simulink model "dpd_pa"  (Simulink 8.7)
settings: Solver=VariableStepDiscrete  StartTime=0.0  StopTime=hepta_dpd_pa_param.endTime  RelTol=1e-3
PreLoadFcn:
  | % Run the setup script when the model is opened
  | setup_dpd_pa;
InitFcn:
  | % Run the setup script again just before the
  | % model is run, so that any updates made
  | % after opening are applied.
  | setup_dpd_pa;
undefined symbols (not defined in the file or in its folder): AdvDSPBChannelOutDisplay, dpoly, dspba_ChannelInVis, dspba_ChannelOutVis, dspba_internal_get_channel_ports, evalAionMaskParam, hepta_dpd_pa_param, latency, value
libraries: DSPBAPrim x159, DSPBABase x6, DSPBAAvalonST x2, DSPBAUtilities x1
(part 1 of 2)
Description:
  | DSP Builder Advanced Template for Template Design implementing Primitive Subsystems
settings Model: Creator=mjervis  LastModifiedBy=5g
settings DataIOCC: SignalLoggingSaveFormat=ModelDataLogs
settings OptimizationCC: ExpressionDepthLimit=2147483647
settings DebuggingCC: SolverPrmCheckMsg=warning  InheritedTsInSrcMsg=none  IntegerOverflowMsg=none  FcnCallInpInsideContextMsg=UseLocalSettings  StateNameClashWarn=warning  IntegerSaturationMsg=none
settings GRTTargetCC: CombineOutputUpdateFcns=off  GRTInterface=on
settings ConfigComp: CovSFcnEnable=off

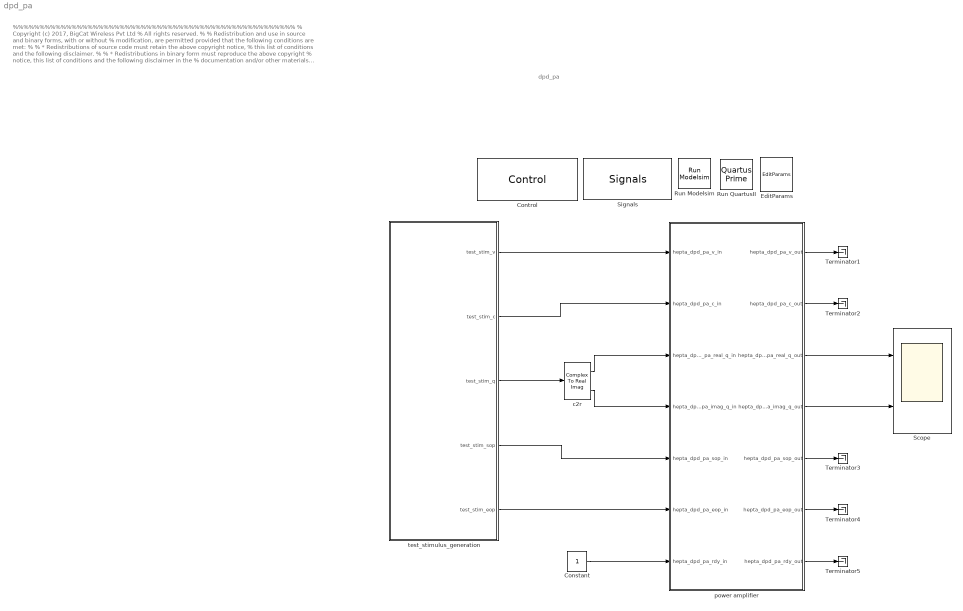
== system dpd_pa ==
  note: %%%%%%%%%%%%%%%%%%%%%%%%%%%%%%%%%%%%%%%%%%%%%%%%%%%%%
      |  % Copyright (c) 2017, BigCat Wireless Pvt Ltd
      |  % All rights reserved.
      |  %
      |  % Redistribution and use in source and binary forms, with or without
      |  % modification, are permitted provided that the following conditions are met:
      |  %
      |  %     * Redistributions of source code must retain the above copyright notice,
      |  %       this list of conditions and the following disclaimer.
      |  %
      |  %     * Redistributions in binary form must reproduce the above copyright
      |  %       notice, this list of conditions and the following disclaimer in the
      |  %       documentation and/or other materials provided with the distribution.
      |  %
      |  %     * Neither the name of the copyright holder nor the names of its contributors
      |  %       may be used to endorse or promote products derived from this software
      |  %       without specific prior written permission.
      |  %
      |  %
      |  %
      |  % THIS SOFTWARE IS PROVIDED BY THE COPYRIGHT HOLDERS AND CONTRIBUTORS "AS IS"
      |  % AND ANY EXPRESS OR IMPLIED WARRANTIES, INCLUDING, BUT NOT LIMITED TO, THE
      |  % IMPLIED WARRANTIES OF MERCHANTABILITY AND FITNESS FOR A PARTICULAR PURPOSE ARE
      |  % DISCLAIMED. IN NO EVENT SHALL THE COPYRIGHT HOLDER OR CONTRIBUTORS BE LIABLE
      |  % FOR ANY DIRECT, INDIRECT, INCIDENTAL, SPECIAL, EXEMPLARY, OR CONSEQUENTIAL
      |  % DAMAGES (INCLUDING, BUT NOT LIMITED TO, PROCUREMENT OF SUBSTITUTE GOODS OR
      |  % SERVICES; LOSS OF USE, DATA, OR PROFITS; OR BUSINESS INTERRUPTION) HOWEVER
      |  % CAUSED AND ON ANY THEORY OF LIABILITY, WHETHER IN CONTRACT, STRICT LIABILITY,
      |  % OR TORT (INCLUDING NEGLIGENCE OR OTHERWISE) ARISING IN ANY WAY OUT OF THE USE
      |  % OF THIS SOFTWARE, EVEN IF ADVISED OF THE POSSIBILITY OF SUCH DAMAGE.
      |  %
      |   %%%%%%%%%%%%%%%%%%%%%%%%%%%%%%%%%%%%%%%%%%%%%%%%%%%%%
  note: dpd_pa
  Constant : Constant  OutDataTypeStr=boolean
  Control : DSPBABase/Control  generate=on  language=VHDL  destination=./rtl  make_full_path=off  path_is_relative=on  autotestbench=on  signaldepth=2  coveragetestbench=on  logs=off  spacewidth=2  spacenum=1  addrwidth=13  datawidth=32  dataendian=Big Endian  hierarchicalnames=off  ramThresholdBits=-1  distRamThresholdBits=-1  mlabThresholdBits=-1  hardMultiplierThresholdLuts=-1  version=20090407  errorOnChanMismatch=1  errorOnGPIOMismatch=0  importModelsimResults=0  cycleAccurate=off  reinterpretCastMult=off  paramFile=dpd_pa_params.xml
  EditParams : DSPBABase/EditParams  version=20090407
  Run Modelsim : DSPBABase/Run Modelsim  version=20090407
  "Run QuartusII " : DSPBABase/Quartus Prime  version=20090407
  Scope : Scope  NumInputPorts=2
  Signals : DSPBABase/Signals  clk=clk  freq=hepta_dpd_pa_param.ClockRate  margin=hepta_dpd_pa_param.ClockMargin  rst=areset  rstactive=High  bus=bus  enbusclock=on  busfreq=61.44  bussync=on  version=20090407
  Terminator{1..5} (5 alike) : Terminator
  c2r : ComplexToRealImag
  power amplifier : Subsystem
  test_stimulus_generation : Subsystem
  wires:
  test_stimulus_generation/1(test_stim_v) -> power amplifier/1(hepta_dpd_pa_v_in)
  test_stimulus_generation/2(test_stim_c) -> power amplifier/2(hepta_dpd_pa_c_in)
  test_stimulus_generation/3(test_stim_q) -> c2r/1
  c2r/1 -> power amplifier/3(hepta_dpd_pa_real_q_in)
  c2r/2 -> power amplifier/4(hepta_dpd_pa_imag_q_in)
  Constant/1 -> power amplifier/7(hepta_dpd_pa_rdy_in)
  power amplifier/1(hepta_dpd_pa_v_out) -> Terminator1/1
  power amplifier/2(hepta_dpd_pa_c_out) -> Terminator2/1
  power amplifier/5(hepta_dpd_pa_sop_out) -> Terminator3/1
  power amplifier/6(hepta_dpd_pa_eop_out) -> Terminator4/1
  power amplifier/7(hepta_dpd_pa_rdy_out) -> Terminator5/1
  power amplifier/3(hepta_dpd_pa_real_q_out) -> Scope/1
  power amplifier/4(hepta_dpd_pa_imag_q_out) -> Scope/2
  test_stimulus_generation/5(test_stim_eop) -> power amplifier/6(hepta_dpd_pa_eop_in)
  test_stimulus_generation/4(test_stim_sop) -> power amplifier/5(hepta_dpd_pa_sop_in)

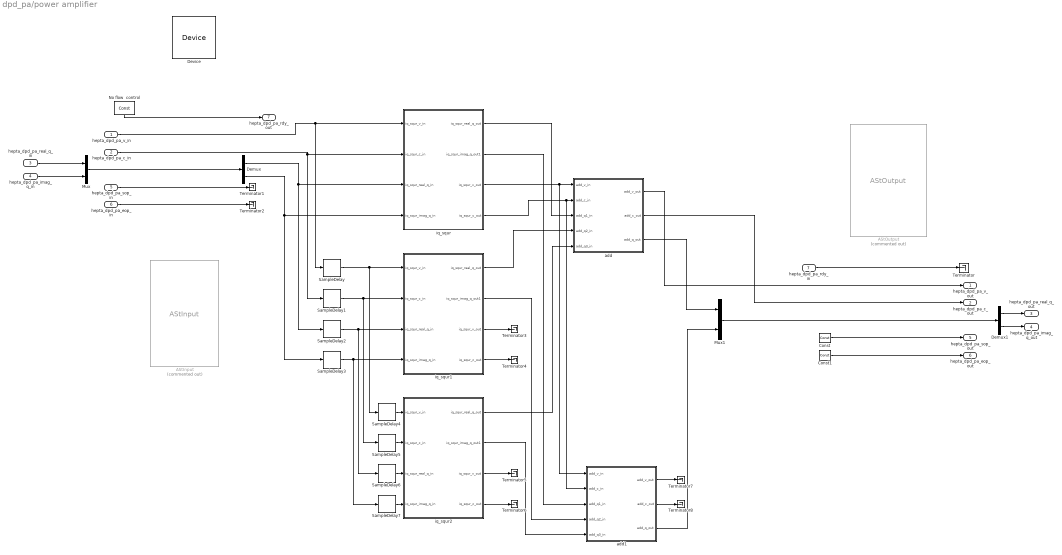
== system dpd_pa/power amplifier ==
  hepta_dpd_pa_v_in : Inport
  hepta_dpd_pa_c_in : Inport  Port=2
  hepta_dpd_pa_real_q_in : Inport  Port=3
  hepta_dpd_pa_imag_q_in : Inport  Port=4
  hepta_dpd_pa_sop_in : Inport  Port=5
  hepta_dpd_pa_eop_in : Inport  Port=6
  hepta_dpd_pa_rdy_in : Inport  Port=7
  AStInput : DSPBAAvalonST/AStInput  Commented=on
      link override BasicAvInput/sopOvrflw/setOrRst1: omode=Inherit via internal rule  otype=ufix(1)  scale=2^0
      link override ChannelOut: value=3  latency=1
  AStOutput : DSPBAAvalonST/AStOutput  Commented=on  fifo_setup=[12 4 8]
      link override ChannelOut: value=4  latency=0
  Const : DSPBAPrim/Const  primtype=const  nInputs=0  nOutputs=1  omode=boolean  otype=sfix(16)  scale=2^-15  rndmethod=Unbiased  factor=1  satmethod=Symmetric  shift_vec=[0 1 2 -1]  value=0  inPortNames=['+'; '+';]  outPortNames=[' ']  dspbaimage=dspba_prim.jpg  text=fprintf('%s', num2str(value));  style=Optimised  visibilities=8 + 1024  floatPrecision=float32_m23  version=20120820
  Const1 : DSPBAPrim/Const  primtype=const  nInputs=0  nOutputs=1  omode=boolean  otype=sfix(16)  scale=2^-15  rndmethod=Unbiased  factor=1  satmethod=Symmetric  shift_vec=[0 1 2 -1]  value=0  inPortNames=['+'; '+';]  outPortNames=[' ']  dspbaimage=dspba_prim.jpg  text=fprintf('%s', num2str(value));  style=Optimised  visibilities=8 + 1024  floatPrecision=float32_m23  version=20120820
  Demux : Demux  Outputs=2
  Demux1 : Demux  Outputs=2
  Device : DSPBABase/Device  family=Arria 10  deviceMember=Arria 10  stratix4device=Stratix IV GX  hardcopy4device=HardCopy IV E  stratix5device=Stratix V GX  device=10AS066N2F40I1SGES  speed=1  stratixSpeed=-5  stratix2Speed=-3  stratix3Speed=-3  stratix4gxSpeed=-2  stratix4gtSpeed=-1  cyclone2Speed=-6  cyclone3Speed=-7  arria2Speed=-4  cyclone4eSpeed=-8  stratix5Speed=-3  arria5Speed=-4  arriaSpeed=-6  cyclone3lsSpeed=-7  cyclone5Speed=-6  arria2gzSpeed=-3  nightFurySpeed=-2  ecp2Speed=-7  hardcopycompat=off  version=20140217  max10flashmode=off  max10nomeminit=off
  Mux : Mux  Inputs=2
  Mux1 : Mux  Inputs=2
  No flow  control : DSPBAPrim/Const  primtype=const  nInputs=0  nOutputs=1  omode=Inherit via internal rule  otype=sfix(16)  scale=2^-15  rndmethod=Unbiased  factor=1  satmethod=Symmetric  shift_vec=[0 1 2 -1]  value=1  inPortNames=['+'; '+';]  outPortNames=[' ']  dspbaimage=dspba_prim.jpg  text=fprintf('%s', num2str(value));  style=Optimised  visibilities=8 + 1024  floatPrecision=float32_m23  version=20120820
  SampleDelay{,1..7} (8 alike) : DSPBAPrim/SampleDelay  primtype=sampdelay  nInputs=1  nOutputs=1  omode=Inherit via internal rule  otype=sfix(16)  scale=2^-15  rndmethod=Unbiased  factor=1  satmethod=Symmetric  shift_vec=[0 1 2 -1]  value=1  inPortNames=[' '; ' ';]  outPortNames=[' ']  dspbaimage=dspba_prim.jpg  text=dpoly(1, eye(1,value+1), 'z')  style=Optimised  visibilities=8 + 1024 + 2^17 + 2^18  flexible=off  slackgroup=0  augmented=0  version=20090407  advOptions=[]
  Terminator{,1..8} (9 alike) : Terminator
  add : Subsystem
  add1 : Subsystem
  iq_squr : Subsystem
  iq_squr1 : Subsystem
  iq_squr2 : Subsystem
  hepta_dpd_pa_v_out : Outport
  hepta_dpd_pa_c_out : Outport  Port=2
  hepta_dpd_pa_real_q_out : Outport  Port=3
  hepta_dpd_pa_imag_q_out : Outport  Port=4
  hepta_dpd_pa_sop_out : Outport  Port=5
  hepta_dpd_pa_eop_out : Outport  Port=6
  hepta_dpd_pa_rdy_out : Outport  Port=7
  wires:
  No flow  control/1 -> hepta_dpd_pa_rdy_out/1
  hepta_dpd_pa_real_q_in/1 -> Mux/1
  hepta_dpd_pa_imag_q_in/1 -> Mux/2
  Mux/1 -> Demux/1
  Demux/2 -> SampleDelay3/1, iq_squr/4(iq_squr_imag_q_in)
  add/1(add_v_out) -> hepta_dpd_pa_v_out/1
  add/2(add_c_out) -> hepta_dpd_pa_c_out/1
  Const/1 -> hepta_dpd_pa_sop_out/1
  Const1/1 -> hepta_dpd_pa_eop_out/1
  hepta_dpd_pa_rdy_in/1 -> Terminator/1
  Mux1/1 -> Demux1/1
  Demux1/2 -> hepta_dpd_pa_imag_q_out/1
  Demux1/1 -> hepta_dpd_pa_real_q_out/1
  hepta_dpd_pa_sop_in/1 -> Terminator1/1
  hepta_dpd_pa_eop_in/1 -> Terminator2/1
  hepta_dpd_pa_v_in/1 -> SampleDelay/1, iq_squr/1(iq_squr_v_in)
  Demux/1 -> SampleDelay2/1, iq_squr/3(iq_squr_real_q_in)
  hepta_dpd_pa_c_in/1 -> SampleDelay1/1, iq_squr/2(iq_squr_c_in)
  SampleDelay/1 -> iq_squr1/1(iq_squr_v_in), SampleDelay4/1
  SampleDelay1/1 -> iq_squr1/2(iq_squr_c_in), SampleDelay5/1
  SampleDelay2/1 -> iq_squr1/3(iq_squr_real_q_in), SampleDelay6/1
  SampleDelay3/1 -> iq_squr1/4(iq_squr_imag_q_in), SampleDelay7/1
  SampleDelay4/1 -> iq_squr2/1(iq_squr_v_in)
  SampleDelay5/1 -> iq_squr2/2(iq_squr_c_in)
  SampleDelay6/1 -> iq_squr2/3(iq_squr_real_q_in)
  SampleDelay7/1 -> iq_squr2/4(iq_squr_imag_q_in)
  iq_squr/3(iq_squr_v_out) -> add1/1(add_v_in), add/1(add_v_in)
  iq_squr/4(iq_squr_c_out) -> add1/2(add_c_in), add/2(add_c_in)
  iq_squr/1(iq_squr_real_q_out) -> add/3(add_q1_in)
  iq_squr1/1(iq_squr_real_q_out) -> add/4(add_q2_in)
  iq_squr2/1(iq_squr_real_q_out) -> add/5(add_q3_in)
  iq_squr2/2(iq_squr_imag_q_out1) -> add1/5(add_q3_in)
  iq_squr1/2(iq_squr_imag_q_out1) -> add1/4(add_q2_in)
  iq_squr/2(iq_squr_imag_q_out1) -> add1/3(add_q1_in)
  add/3(add_q_out) -> Mux1/1
  add1/3(add_q_out) -> Mux1/2
  iq_squr1/3(iq_squr_v_out) -> Terminator3/1
  iq_squr1/4(iq_squr_c_out) -> Terminator4/1
  iq_squr2/3(iq_squr_v_out) -> Terminator5/1
  iq_squr2/4(iq_squr_c_out) -> Terminator6/1
  add1/1(add_v_out) -> Terminator7/1
  add1/2(add_c_out) -> Terminator8/1

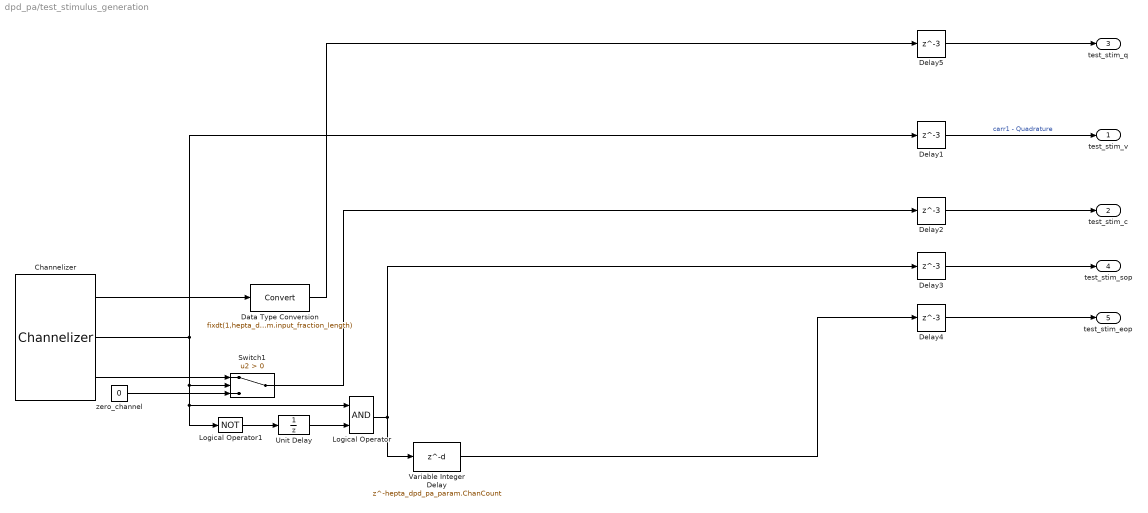
== system dpd_pa/test_stimulus_generation ==
  Channelizer : DSPBAUtilities/Channelizer  data_input=hepta_dpd_pa_param.inputdata1  folding=hepta_dpd_pa_param.Period  samples_valid=1  samples_idle=0  sample_time=hepta_dpd_pa_param.SampleTime
  Data Type Conversion : DataTypeConversion  OutDataTypeStr=fixdt(1,hepta_dpd_pa_param.input_word_length,hepta_dpd_pa_param.input_fraction_length)  SaturateOnIntegerOverflow=on
  Delay{1..4} (4 alike) : Delay  DelayLength=3  InitialCondition=0
  Delay5 : Delay  DelayLength=3  InitialCondition=0  InputProcessing=Inherited
  Logical Operator : Logic  AllPortsSameDT=off  OutDataTypeStr=boolean
  Logical Operator1 : Logic  Operator=NOT  AllPortsSameDT=off  OutDataTypeStr=boolean
  Switch1 : Switch  Criteria=u2 > Threshold
  Unit Delay : UnitDelay  SampleTime=-1
  Variable Integer Delay : Delay  DelayLength=hepta_dpd_pa_param.ChanCount  InputProcessing=Inherited
  zero_channel : Constant  Value=0  OutDataTypeStr=uint8
  test_stim_v : Outport
  test_stim_c : Outport  Port=2
  test_stim_q : Outport  Port=3
  test_stim_sop : Outport  Port=4
  test_stim_eop : Outport  Port=5
  wires:
  Channelizer/3 -> Switch1/1
  Logical Operator1/1 -> Unit Delay/1
  Channelizer/1 -> Data Type Conversion/1
  Logical Operator/1 -> Variable Integer Delay/1, Delay3/1
  zero_channel/1 -> Switch1/3
  Unit Delay/1 -> Logical Operator/2
  Channelizer/2 -> Logical Operator/1, Logical Operator1/1, Switch1/2, Delay1/1
  Switch1/1 -> Delay2/1
  Variable Integer Delay/1 -> Delay4/1
  Delay2/1 -> test_stim_c/1
  Delay3/1 -> test_stim_sop/1
  Delay4/1 -> test_stim_eop/1
  Delay1/1 -> test_stim_v/1  "carr1 - Quadrature"
  Data Type Conversion/1 -> Delay5/1
  Delay5/1 -> test_stim_q/1

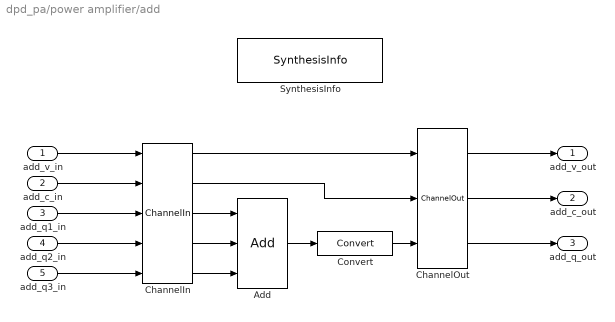
== system dpd_pa/power amplifier/add ==
  add_v_in : Inport
  add_c_in : Inport  Port=2
  add_q1_in : Inport  Port=3
  add_q2_in : Inport  Port=4
  add_q3_in : Inport  Port=5
  Add : DSPBAPrim/Add  primtype=add  nInputs=evalAionMaskParam(gcb,'value',1)  nOutputs=1  omode=Inherit via internal rule with word growth  otype=sfix(16)  scale=2^-15  rndmethod=Unbiased  factor=1  satmethod=Symmetric  shift_vec=[0 1 2 -1]  value=3  inPortNames=[' '; ' ';]  outPortNames=[' ']  dspbaimage=dspba_prim.jpg  text=fprintf('+');  style=Optimised  visibilities=1032+2^17+2^18+2^19  genFPC=off  floatRounding=correct  advOptions=[]  version=20130821
  ChannelIn : DSPBAPrim/ChannelIn  primtype=channelin  nInputs=dspba_internal_get_channel_ports(gcb)  nOutputs=dspba_internal_get_channel_ports(gcb)  omode=Inherit via internal rule  otype=sfix(16)  scale=2^-15  rndmethod=Unbiased  factor=1  satmethod=Symmetric  shift_vec=[0 1 2 -1]  value=3  inPortNames=['v'; 'c'; '0'; '1'; '2'; '3'; '4'; '5'; '6'; '7'; '8'; '9'; 'A'; 'B'; 'D'; 'E'; 'F'; 'G'; 'H'; 'I'; 'J'; 'K'; 'L'; 'M'; 'N'; 'O'; 'P'; 'Q'; 'R'; 'S'; 'T'; 'U'; 'W'; 'X'; 'Y'; 'Z']  outPortNames=['v'; 'c'; '0'; '1'; '2'; '3'; '4'; '5'; '6'; '7'; '8'; '9'; 'A'; 'B'; 'D'; 'E'; 'F'; 'G'; 'H'; 'I'; 'J'; 'K'; 'L'; 'M'; 'N'; 'O'; 'P'; 'Q'; 'R'; 'S'; 'T'; 'U'; 'W'; 'X'; 'Y'; 'Z']  dspbaimage=dspba_prim.jpg  text=fprintf('In');  style=Optimised  dataSignals=3  foldingEnabled=off  channels=1  sampleRate=200  packetBeginPresent=off  packetBeginEnabled=off  visibilities=dspba_ChannelInVis(gcb)  latencyCorrection=0  version=20141013
  ChannelOut : DSPBAPrim/ChannelOut  primtype=channelout  nInputs=dspba_internal_get_channel_ports(gcb)  nOutputs=dspba_internal_get_channel_ports(gcb)  omode=Inherit via internal rule  otype=sfix(16)  scale=2^-15  rndmethod=Unbiased  factor=1  satmethod=Symmetric  shift_vec=[0 1 2 -1]  value=1  inPortNames=['v'; 'c'; '0'; '1'; '2'; '3'; '4'; '5'; '6'; '7'; '8'; '9'; 'A'; 'B'; 'D'; 'E'; 'F'; 'G'; 'H'; 'I'; 'J'; 'K'; 'L'; 'M'; 'N'; 'O'; 'P'; 'Q'; 'R'; 'S'; 'T'; 'U'; 'W'; 'X'; 'Y'; 'Z']  outPortNames=['v'; 'c'; '0'; '1'; '2'; '3'; '4'; '5'; '6'; '7'; '8'; '9'; 'A'; 'B'; 'D'; 'E'; 'F'; 'G'; 'H'; 'I'; 'J'; 'K'; 'L'; 'M'; 'N'; 'O'; 'P'; 'Q'; 'R'; 'S'; 'T'; 'U'; 'W'; 'X'; 'Y'; 'Z']  dspbaimage=dspba_prim.jpg  text=fprintf('Out%s', AdvDSPBChannelOutDisplay(latency));  style=Optimised  dataSignals=1  foldingEnabled=off  channels=1  sampleRate=200  packetBeginPresent=off  packetBeginEnabled=off  visibilities=dspba_ChannelOutVis(gcb)  latency=0  latencyCorrection=0  version=20141013
  Convert : DSPBAPrim/Convert  primtype=convert  nInputs=1  nOutputs=1  omode=Specify via dialog  otype=sfix(16)  scale=2^-15  rndmethod=Unbiased  factor=1  satmethod=None  shift_vec=[0 1 2 -1]  value=round([0:255]/17)  inPortNames=[' '; ' ';]  outPortNames=[' '; 'c']  dspbaimage=dspba_prim.jpg  text=fprintf('convert');  style=Optimised  visibilities=8+64+256+2^17  clipdetect=off  floatPrecision=float32_m23  advOptions=[]  version=20130211
  SynthesisInfo : DSPBAPrim/SynthesisInfo  primtype=synthinfo  nInputs=0  nOutputs=0  omode=Inherit via internal rule  otype=sfix(16)  scale=2^-15  rndmethod=Truncate  factor=1  satmethod=Symmetric  shift_vec=[0 1 2 -1]  value=99  inPortNames=[' '; ' ';]  outPortNames=[' ']  dspbaimage=dspba_prim_ctrl.jpg  text=fprintf('Style=%s', style);  style=Scheduled  visibilities=2^15+2^17+2^18+2^19  constraintInUse=off  constraintRelation=>  constraintLimit=2  bitAccurate=off  version=20150220
  add_v_out : Outport
  add_c_out : Outport  Port=2
  add_q_out : Outport  Port=3
  wires:
  ChannelIn/1 -> ChannelOut/1
  add_c_in/1 -> ChannelIn/2
  add_q1_in/1 -> ChannelIn/3
  add_v_in/1 -> ChannelIn/1
  add_q2_in/1 -> ChannelIn/4
  add_q3_in/1 -> ChannelIn/5
  ChannelIn/2 -> ChannelOut/2
  ChannelOut/2 -> add_c_out/1
  Add/1 -> Convert/1
  ChannelOut/1 -> add_v_out/1
  ChannelOut/3 -> add_q_out/1
  ChannelIn/3 -> Add/1
  ChannelIn/4 -> Add/2
  ChannelIn/5 -> Add/3
  Convert/1 -> ChannelOut/3

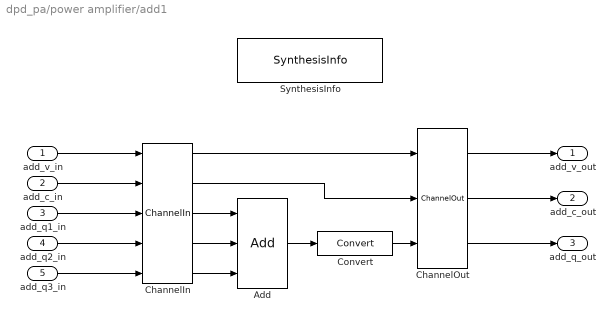
== system dpd_pa/power amplifier/add1 ==
  add_v_in : Inport
  add_c_in : Inport  Port=2
  add_q1_in : Inport  Port=3
  add_q2_in : Inport  Port=4
  add_q3_in : Inport  Port=5
  Add : DSPBAPrim/Add  primtype=add  nInputs=evalAionMaskParam(gcb,'value',1)  nOutputs=1  omode=Inherit via internal rule with word growth  otype=sfix(16)  scale=2^-15  rndmethod=Unbiased  factor=1  satmethod=Symmetric  shift_vec=[0 1 2 -1]  value=3  inPortNames=[' '; ' ';]  outPortNames=[' ']  dspbaimage=dspba_prim.jpg  text=fprintf('+');  style=Optimised  visibilities=1032+2^17+2^18+2^19  genFPC=off  floatRounding=correct  advOptions=[]  version=20130821
  ChannelIn : DSPBAPrim/ChannelIn  primtype=channelin  nInputs=dspba_internal_get_channel_ports(gcb)  nOutputs=dspba_internal_get_channel_ports(gcb)  omode=Inherit via internal rule  otype=sfix(16)  scale=2^-15  rndmethod=Unbiased  factor=1  satmethod=Symmetric  shift_vec=[0 1 2 -1]  value=3  inPortNames=['v'; 'c'; '0'; '1'; '2'; '3'; '4'; '5'; '6'; '7'; '8'; '9'; 'A'; 'B'; 'D'; 'E'; 'F'; 'G'; 'H'; 'I'; 'J'; 'K'; 'L'; 'M'; 'N'; 'O'; 'P'; 'Q'; 'R'; 'S'; 'T'; 'U'; 'W'; 'X'; 'Y'; 'Z']  outPortNames=['v'; 'c'; '0'; '1'; '2'; '3'; '4'; '5'; '6'; '7'; '8'; '9'; 'A'; 'B'; 'D'; 'E'; 'F'; 'G'; 'H'; 'I'; 'J'; 'K'; 'L'; 'M'; 'N'; 'O'; 'P'; 'Q'; 'R'; 'S'; 'T'; 'U'; 'W'; 'X'; 'Y'; 'Z']  dspbaimage=dspba_prim.jpg  text=fprintf('In');  style=Optimised  dataSignals=3  foldingEnabled=off  channels=1  sampleRate=200  packetBeginPresent=off  packetBeginEnabled=off  visibilities=dspba_ChannelInVis(gcb)  latencyCorrection=0  version=20141013
  ChannelOut : DSPBAPrim/ChannelOut  primtype=channelout  nInputs=dspba_internal_get_channel_ports(gcb)  nOutputs=dspba_internal_get_channel_ports(gcb)  omode=Inherit via internal rule  otype=sfix(16)  scale=2^-15  rndmethod=Unbiased  factor=1  satmethod=Symmetric  shift_vec=[0 1 2 -1]  value=1  inPortNames=['v'; 'c'; '0'; '1'; '2'; '3'; '4'; '5'; '6'; '7'; '8'; '9'; 'A'; 'B'; 'D'; 'E'; 'F'; 'G'; 'H'; 'I'; 'J'; 'K'; 'L'; 'M'; 'N'; 'O'; 'P'; 'Q'; 'R'; 'S'; 'T'; 'U'; 'W'; 'X'; 'Y'; 'Z']  outPortNames=['v'; 'c'; '0'; '1'; '2'; '3'; '4'; '5'; '6'; '7'; '8'; '9'; 'A'; 'B'; 'D'; 'E'; 'F'; 'G'; 'H'; 'I'; 'J'; 'K'; 'L'; 'M'; 'N'; 'O'; 'P'; 'Q'; 'R'; 'S'; 'T'; 'U'; 'W'; 'X'; 'Y'; 'Z']  dspbaimage=dspba_prim.jpg  text=fprintf('Out%s', AdvDSPBChannelOutDisplay(latency));  style=Optimised  dataSignals=1  foldingEnabled=off  channels=1  sampleRate=200  packetBeginPresent=off  packetBeginEnabled=off  visibilities=dspba_ChannelOutVis(gcb)  latency=0  latencyCorrection=0  version=20141013
  Convert : DSPBAPrim/Convert  primtype=convert  nInputs=1  nOutputs=1  omode=Specify via dialog  otype=sfix(16)  scale=2^-15  rndmethod=Unbiased  factor=1  satmethod=None  shift_vec=[0 1 2 -1]  value=round([0:255]/17)  inPortNames=[' '; ' ';]  outPortNames=[' '; 'c']  dspbaimage=dspba_prim.jpg  text=fprintf('convert');  style=Optimised  visibilities=8+64+256+2^17  clipdetect=off  floatPrecision=float32_m23  advOptions=[]  version=20130211
  SynthesisInfo : DSPBAPrim/SynthesisInfo  primtype=synthinfo  nInputs=0  nOutputs=0  omode=Inherit via internal rule  otype=sfix(16)  scale=2^-15  rndmethod=Truncate  factor=1  satmethod=Symmetric  shift_vec=[0 1 2 -1]  value=99  inPortNames=[' '; ' ';]  outPortNames=[' ']  dspbaimage=dspba_prim_ctrl.jpg  text=fprintf('Style=%s', style);  style=Scheduled  visibilities=2^15+2^17+2^18+2^19  constraintInUse=off  constraintRelation=>  constraintLimit=2  bitAccurate=off  version=20150220
  add_v_out : Outport
  add_c_out : Outport  Port=2
  add_q_out : Outport  Port=3
  wires:
  ChannelIn/1 -> ChannelOut/1
  add_c_in/1 -> ChannelIn/2
  add_q1_in/1 -> ChannelIn/3
  add_v_in/1 -> ChannelIn/1
  add_q2_in/1 -> ChannelIn/4
  add_q3_in/1 -> ChannelIn/5
  ChannelIn/2 -> ChannelOut/2
  ChannelOut/2 -> add_c_out/1
  Add/1 -> Convert/1
  ChannelOut/1 -> add_v_out/1
  ChannelOut/3 -> add_q_out/1
  ChannelIn/3 -> Add/1
  ChannelIn/4 -> Add/2
  ChannelIn/5 -> Add/3
  Convert/1 -> ChannelOut/3

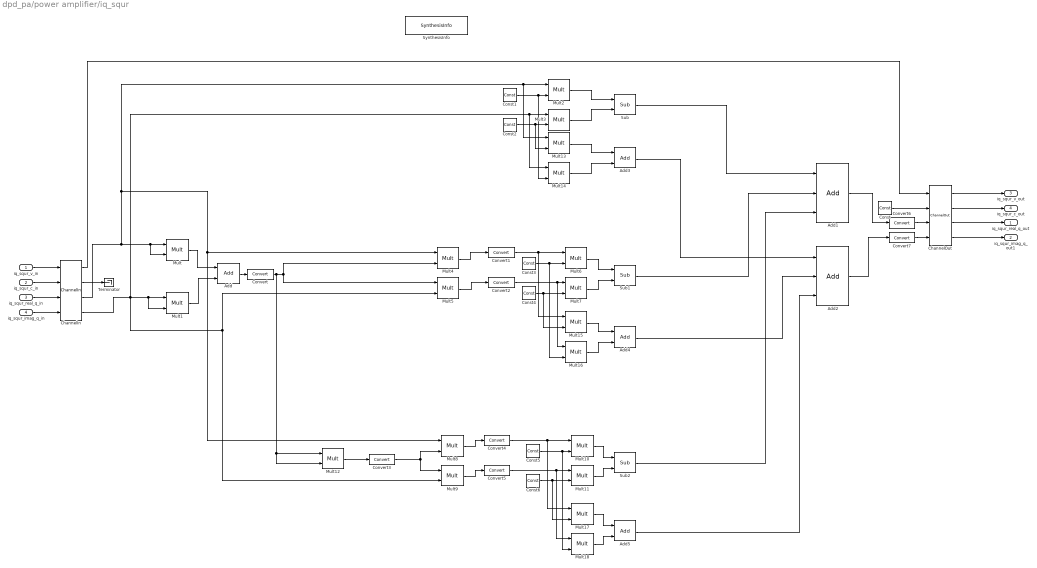
== system dpd_pa/power amplifier/iq_squr ==
  iq_squr_v_in : Inport
  iq_squr_c_in : Inport  Port=2
  iq_squr_real_q_in : Inport  Port=3
  iq_squr_imag_q_in : Inport  Port=4
  Add{,3..5} (4 alike) : DSPBAPrim/Add  primtype=add  nInputs=evalAionMaskParam(gcb,'value',1)  nOutputs=1  omode=Inherit via internal rule with word growth  otype=sfix(16)  scale=2^-15  rndmethod=Unbiased  factor=1  satmethod=Symmetric  shift_vec=[0 1 2 -1]  value=2  inPortNames=[' '; ' ';]  outPortNames=[' ']  dspbaimage=dspba_prim.jpg  text=fprintf('+');  style=Optimised  visibilities=1032+2^17+2^18+2^19  genFPC=off  floatRounding=correct  advOptions=[]  version=20130821
  Add1 : DSPBAPrim/Add  primtype=add  nInputs=evalAionMaskParam(gcb,'value',1)  nOutputs=1  omode=Inherit via internal rule with word growth  otype=sfix(16)  scale=2^-15  rndmethod=Unbiased  factor=1  satmethod=Symmetric  shift_vec=[0 1 2 -1]  value=3  inPortNames=[' '; ' ';]  outPortNames=[' ']  dspbaimage=dspba_prim.jpg  text=fprintf('+');  style=Optimised  visibilities=1032+2^17+2^18+2^19  genFPC=off  floatRounding=correct  advOptions=[]  version=20130821
  Add2 : DSPBAPrim/Add  primtype=add  nInputs=evalAionMaskParam(gcb,'value',1)  nOutputs=1  omode=Inherit via internal rule with word growth  otype=sfix(16)  scale=2^-15  rndmethod=Unbiased  factor=1  satmethod=Symmetric  shift_vec=[0 1 2 -1]  value=3  inPortNames=[' '; ' ';]  outPortNames=[' ']  dspbaimage=dspba_prim.jpg  text=fprintf('+');  style=Optimised  visibilities=1032+2^17+2^18+2^19  genFPC=off  floatRounding=correct  advOptions=[]  version=20130821
  ChannelIn : DSPBAPrim/ChannelIn  primtype=channelin  nInputs=dspba_internal_get_channel_ports(gcb)  nOutputs=dspba_internal_get_channel_ports(gcb)  omode=Inherit via internal rule  otype=sfix(16)  scale=2^-15  rndmethod=Unbiased  factor=1  satmethod=Symmetric  shift_vec=[0 1 2 -1]  value=2  inPortNames=['v'; 'c'; '0'; '1'; '2'; '3'; '4'; '5'; '6'; '7'; '8'; '9'; 'A'; 'B'; 'D'; 'E'; 'F'; 'G'; 'H'; 'I'; 'J'; 'K'; 'L'; 'M'; 'N'; 'O'; 'P'; 'Q'; 'R'; 'S'; 'T'; 'U'; 'W'; 'X'; 'Y'; 'Z']  outPortNames=['v'; 'c'; '0'; '1'; '2'; '3'; '4'; '5'; '6'; '7'; '8'; '9'; 'A'; 'B'; 'D'; 'E'; 'F'; 'G'; 'H'; 'I'; 'J'; 'K'; 'L'; 'M'; 'N'; 'O'; 'P'; 'Q'; 'R'; 'S'; 'T'; 'U'; 'W'; 'X'; 'Y'; 'Z']  dspbaimage=dspba_prim.jpg  text=fprintf('In');  style=Optimised  dataSignals=2  foldingEnabled=off  channels=1  sampleRate=200  packetBeginPresent=off  packetBeginEnabled=off  visibilities=dspba_ChannelInVis(gcb)  latencyCorrection=0  version=20141013
  ChannelOut : DSPBAPrim/ChannelOut  primtype=channelout  nInputs=dspba_internal_get_channel_ports(gcb)  nOutputs=dspba_internal_get_channel_ports(gcb)  omode=Inherit via internal rule  otype=sfix(16)  scale=2^-15  rndmethod=Unbiased  factor=1  satmethod=Symmetric  shift_vec=[0 1 2 -1]  value=2  inPortNames=['v'; 'c'; '0'; '1'; '2'; '3'; '4'; '5'; '6'; '7'; '8'; '9'; 'A'; 'B'; 'D'; 'E'; 'F'; 'G'; 'H'; 'I'; 'J'; 'K'; 'L'; 'M'; 'N'; 'O'; 'P'; 'Q'; 'R'; 'S'; 'T'; 'U'; 'W'; 'X'; 'Y'; 'Z']  outPortNames=['v'; 'c'; '0'; '1'; '2'; '3'; '4'; '5'; '6'; '7'; '8'; '9'; 'A'; 'B'; 'D'; 'E'; 'F'; 'G'; 'H'; 'I'; 'J'; 'K'; 'L'; 'M'; 'N'; 'O'; 'P'; 'Q'; 'R'; 'S'; 'T'; 'U'; 'W'; 'X'; 'Y'; 'Z']  dspbaimage=dspba_prim.jpg  text=fprintf('Out%s', AdvDSPBChannelOutDisplay(latency));  style=Optimised  dataSignals=2  foldingEnabled=off  channels=1  sampleRate=200  packetBeginPresent=off  packetBeginEnabled=off  visibilities=dspba_ChannelOutVis(gcb)  latency=15  latencyCorrection=0  version=20141013
  Const : DSPBAPrim/Const  primtype=const  nInputs=0  nOutputs=1  omode=Specify via dialog  otype=uint(8)  scale=0  rndmethod=Unbiased  factor=1  satmethod=Symmetric  shift_vec=[0 1 2 -1]  value=0  inPortNames=['+'; '+';]  outPortNames=[' ']  dspbaimage=dspba_prim.jpg  text=fprintf('%s', num2str(value));  style=Optimised  visibilities=8 + 1024  floatPrecision=float32_m23  version=20120820
  Const1 : DSPBAPrim/Const  primtype=const  nInputs=0  nOutputs=1  omode=Specify via dialog  otype=sfix(16)  scale=2^-14  rndmethod=Unbiased  factor=1  satmethod=Symmetric  shift_vec=[0 1 2 -1]  value=17225  inPortNames=['+'; '+';]  outPortNames=[' ']  dspbaimage=dspba_prim.jpg  text=fprintf('%s', num2str(value));  style=Optimised  visibilities=8 + 1024  floatPrecision=float32_m23  version=20120820
  Const2 : DSPBAPrim/Const  primtype=const  nInputs=0  nOutputs=1  omode=Specify via dialog  otype=sfix(16)  scale=2^-15  rndmethod=Unbiased  factor=1  satmethod=Symmetric  shift_vec=[0 1 2 -1]  value=2962  inPortNames=['+'; '+';]  outPortNames=[' ']  dspbaimage=dspba_prim.jpg  text=fprintf('%s', num2str(value));  style=Optimised  visibilities=8 + 1024  floatPrecision=float32_m23  version=20120820
  Const3 : DSPBAPrim/Const  primtype=const  nInputs=0  nOutputs=1  omode=Specify via dialog  otype=sfix(16)  scale=2^-15  rndmethod=Unbiased  factor=1  satmethod=Symmetric  shift_vec=[0 1 2 -1]  value=63760  inPortNames=['+'; '+';]  outPortNames=[' ']  dspbaimage=dspba_prim.jpg  text=fprintf('%s', num2str(value));  style=Optimised  visibilities=8 + 1024  floatPrecision=float32_m23  version=20120820
  Const4 : DSPBAPrim/Const  primtype=const  nInputs=0  nOutputs=1  omode=Specify via dialog  otype=sfix(16)  scale=2^-15  rndmethod=Unbiased  factor=1  satmethod=Symmetric  shift_vec=[0 1 2 -1]  value=9503  inPortNames=['+'; '+';]  outPortNames=[' ']  dspbaimage=dspba_prim.jpg  text=fprintf('%s', num2str(value));  style=Optimised  visibilities=8 + 1024  floatPrecision=float32_m23  version=20120820
  Const5 : DSPBAPrim/Const  primtype=const  nInputs=0  nOutputs=1  omode=Specify via dialog  otype=sfix(16)  scale=2^-15  rndmethod=Unbiased  factor=1  satmethod=Symmetric  shift_vec=[0 1 2 -1]  value=33892  inPortNames=['+'; '+';]  outPortNames=[' ']  dspbaimage=dspba_prim.jpg  text=fprintf('%s', num2str(value));  style=Optimised  visibilities=8 + 1024  floatPrecision=float32_m23  version=20120820
  Const6 : DSPBAPrim/Const  primtype=const  nInputs=0  nOutputs=1  omode=Specify via dialog  otype=sfix(16)  scale=2^-15  rndmethod=Unbiased  factor=1  satmethod=Symmetric  shift_vec=[0 1 2 -1]  value=42507  inPortNames=['+'; '+';]  outPortNames=[' ']  dspbaimage=dspba_prim.jpg  text=fprintf('%s', num2str(value));  style=Optimised  visibilities=8 + 1024  floatPrecision=float32_m23  version=20120820
  Convert{,1..7} (8 alike) : DSPBAPrim/Convert  primtype=convert  nInputs=1  nOutputs=1  omode=Specify via dialog  otype=sfix(16)  scale=2^-15  rndmethod=Unbiased  factor=1  satmethod=None  shift_vec=[0 1 2 -1]  value=round([0:255]/17)  inPortNames=[' '; ' ';]  outPortNames=[' '; 'c']  dspbaimage=dspba_prim.jpg  text=fprintf('convert');  style=Optimised  visibilities=8+64+256+2^17  clipdetect=off  floatPrecision=float32_m23  advOptions=[]  version=20130211
  Mult{,1..18} (19 alike) : DSPBAPrim/Mult  primtype=mult  nInputs=2  nOutputs=1  omode=Inherit via internal rule  otype=sfix(16)  scale=2^-15  rndmethod=Unbiased  factor=1  satmethod=Symmetric  shift_vec=[0 1 2 -1]  value=0  inPortNames=[' '; ' ';]  outPortNames=[' ']  dspbaimage=dspba_prim.jpg  text=fprintf('X');  style=Optimised  visibilities=8+2^18+2^19  floatPrecision=float32_m23  floatRounding=correct  advOptions=[]  version=20130115
  Sub : DSPBAPrim/Sub  primtype=sub  nInputs=2  nOutputs=1  omode=Inherit via internal rule with word growth  otype=sfix(16)  scale=2^-15  rndmethod=Unbiased  factor=1  satmethod=Symmetric  shift_vec=[0 1 2 -1]  value=0  inPortNames=['+'; '-';]  outPortNames=[' ']  dspbaimage=dspba_prim.jpg  text=fprintf('-');  style=Optimised  visibilities=8+2^17+2^18  floatRounding=correct  advOptions=[]  version=20130115
  Sub1 : DSPBAPrim/Sub  primtype=sub  nInputs=2  nOutputs=1  omode=Inherit via internal rule with word growth  otype=sfix(16)  scale=2^-15  rndmethod=Unbiased  factor=1  satmethod=Symmetric  shift_vec=[0 1 2 -1]  value=0  inPortNames=['+'; '-';]  outPortNames=[' ']  dspbaimage=dspba_prim.jpg  text=fprintf('-');  style=Optimised  visibilities=8+2^17+2^18  floatRounding=correct  advOptions=[]  version=20130115
  Sub2 : DSPBAPrim/Sub  primtype=sub  nInputs=2  nOutputs=1  omode=Inherit via internal rule with word growth  otype=sfix(16)  scale=2^-15  rndmethod=Unbiased  factor=1  satmethod=Symmetric  shift_vec=[0 1 2 -1]  value=0  inPortNames=['+'; '-';]  outPortNames=[' ']  dspbaimage=dspba_prim.jpg  text=fprintf('-');  style=Optimised  visibilities=8+2^17+2^18  floatRounding=correct  advOptions=[]  version=20130115
  SynthesisInfo : DSPBAPrim/SynthesisInfo  primtype=synthinfo  nInputs=0  nOutputs=0  omode=Inherit via internal rule  otype=sfix(16)  scale=2^-15  rndmethod=Truncate  factor=1  satmethod=Symmetric  shift_vec=[0 1 2 -1]  value=99  inPortNames=[' '; ' ';]  outPortNames=[' ']  dspbaimage=dspba_prim_ctrl.jpg  text=fprintf('Style=%s', style);  style=Scheduled  visibilities=2^15+2^17+2^18+2^19  constraintInUse=off  constraintRelation=>  constraintLimit=2  bitAccurate=off  version=20150220
  Terminator : Terminator
  iq_squr_real_q_out : Outport
  iq_squr_imag_q_out1 : Outport  Port=2
  iq_squr_v_out : Outport  Port=3
  iq_squr_c_out : Outport  Port=4
  wires:
  Mult/1 -> Add/1
  Mult1/1 -> Add/2
  iq_squr_imag_q_in/1 -> ChannelIn/4
  iq_squr_real_q_in/1 -> ChannelIn/3
  ChannelOut/3 -> iq_squr_real_q_out/1
  ChannelOut/1 -> iq_squr_v_out/1
  ChannelOut/2 -> iq_squr_c_out/1
  iq_squr_v_in/1 -> ChannelIn/1
  iq_squr_c_in/1 -> ChannelIn/2
  ChannelIn/2 -> Terminator/1
  ChannelIn/3 -> Mult13/1, Mult2/1, Mult8/1, Mult4/1, Mult/2, Mult/1
  ChannelIn/4 -> Mult14/1, Mult3/1, Mult5/2, Mult9/2, Mult1/2, Mult1/1
  Const/1 -> ChannelOut/2
  Add/1 -> Convert/1
  Const3/1 -> Mult16/2, Mult6/2
  Const4/1 -> Mult15/2, Mult7/2
  Mult4/1 -> Convert1/1
  Mult5/1 -> Convert2/1
  Const5/1 -> Mult18/2, Mult10/2
  Const6/1 -> Mult17/2, Mult11/2
  Mult8/1 -> Convert4/1
  Mult9/1 -> Convert5/1
  Mult12/1 -> Convert3/1
  Convert/1 -> Mult12/2, Mult12/1, Mult5/1, Mult4/2
  Convert1/1 -> Mult15/1, Mult6/1
  Convert2/1 -> Mult16/1, Mult7/1
  Convert3/1 -> Mult9/1, Mult8/2
  Convert4/1 -> Mult17/1, Mult10/1
  Convert5/1 -> Mult18/1, Mult11/1
  Add1/1 -> Convert6/1
  Add2/1 -> Convert7/1
  ChannelIn/1 -> ChannelOut/1
  Convert6/1 -> ChannelOut/3
  Convert7/1 -> ChannelOut/4
  ChannelOut/4 -> iq_squr_imag_q_out1/1
  Const1/1 -> Mult14/2, Mult2/2
  Const2/1 -> Mult13/2, Mult3/2
  Mult2/1 -> Sub/1
  Mult3/1 -> Sub/2
  Mult13/1 -> Add3/1
  Mult14/1 -> Add3/2
  Sub/1 -> Add1/1
  Add3/1 -> Add2/1
  Mult6/1 -> Sub1/1
  Mult7/1 -> Sub1/2
  Mult15/1 -> Add4/1
  Mult16/1 -> Add4/2
  Sub1/1 -> Add1/2
  Add4/1 -> Add2/2
  Mult10/1 -> Sub2/1
  Mult11/1 -> Sub2/2
  Mult17/1 -> Add5/1
  Mult18/1 -> Add5/2
  Add5/1 -> Add2/3
  Sub2/1 -> Add1/3

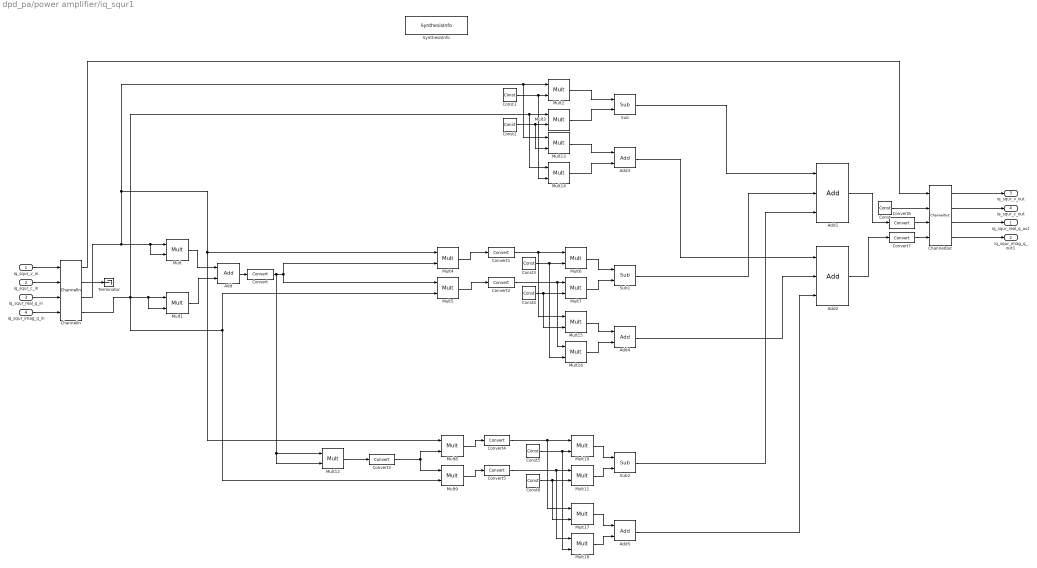
== system dpd_pa/power amplifier/iq_squr1 ==
  iq_squr_v_in : Inport
  iq_squr_c_in : Inport  Port=2
  iq_squr_real_q_in : Inport  Port=3
  iq_squr_imag_q_in : Inport  Port=4
  Add{,3..5} (4 alike) : DSPBAPrim/Add  primtype=add  nInputs=evalAionMaskParam(gcb,'value',1)  nOutputs=1  omode=Inherit via internal rule with word growth  otype=sfix(16)  scale=2^-15  rndmethod=Unbiased  factor=1  satmethod=Symmetric  shift_vec=[0 1 2 -1]  value=2  inPortNames=[' '; ' ';]  outPortNames=[' ']  dspbaimage=dspba_prim.jpg  text=fprintf('+');  style=Optimised  visibilities=1032+2^17+2^18+2^19  genFPC=off  floatRounding=correct  advOptions=[]  version=20130821
  Add1 : DSPBAPrim/Add  primtype=add  nInputs=evalAionMaskParam(gcb,'value',1)  nOutputs=1  omode=Inherit via internal rule with word growth  otype=sfix(16)  scale=2^-15  rndmethod=Unbiased  factor=1  satmethod=Symmetric  shift_vec=[0 1 2 -1]  value=3  inPortNames=[' '; ' ';]  outPortNames=[' ']  dspbaimage=dspba_prim.jpg  text=fprintf('+');  style=Optimised  visibilities=1032+2^17+2^18+2^19  genFPC=off  floatRounding=correct  advOptions=[]  version=20130821
  Add2 : DSPBAPrim/Add  primtype=add  nInputs=evalAionMaskParam(gcb,'value',1)  nOutputs=1  omode=Inherit via internal rule with word growth  otype=sfix(16)  scale=2^-15  rndmethod=Unbiased  factor=1  satmethod=Symmetric  shift_vec=[0 1 2 -1]  value=3  inPortNames=[' '; ' ';]  outPortNames=[' ']  dspbaimage=dspba_prim.jpg  text=fprintf('+');  style=Optimised  visibilities=1032+2^17+2^18+2^19  genFPC=off  floatRounding=correct  advOptions=[]  version=20130821
  ChannelIn : DSPBAPrim/ChannelIn  primtype=channelin  nInputs=dspba_internal_get_channel_ports(gcb)  nOutputs=dspba_internal_get_channel_ports(gcb)  omode=Inherit via internal rule  otype=sfix(16)  scale=2^-15  rndmethod=Unbiased  factor=1  satmethod=Symmetric  shift_vec=[0 1 2 -1]  value=2  inPortNames=['v'; 'c'; '0'; '1'; '2'; '3'; '4'; '5'; '6'; '7'; '8'; '9'; 'A'; 'B'; 'D'; 'E'; 'F'; 'G'; 'H'; 'I'; 'J'; 'K'; 'L'; 'M'; 'N'; 'O'; 'P'; 'Q'; 'R'; 'S'; 'T'; 'U'; 'W'; 'X'; 'Y'; 'Z']  outPortNames=['v'; 'c'; '0'; '1'; '2'; '3'; '4'; '5'; '6'; '7'; '8'; '9'; 'A'; 'B'; 'D'; 'E'; 'F'; 'G'; 'H'; 'I'; 'J'; 'K'; 'L'; 'M'; 'N'; 'O'; 'P'; 'Q'; 'R'; 'S'; 'T'; 'U'; 'W'; 'X'; 'Y'; 'Z']  dspbaimage=dspba_prim.jpg  text=fprintf('In');  style=Optimised  dataSignals=2  foldingEnabled=off  channels=1  sampleRate=200  packetBeginPresent=off  packetBeginEnabled=off  visibilities=dspba_ChannelInVis(gcb)  latencyCorrection=0  version=20141013
  ChannelOut : DSPBAPrim/ChannelOut  primtype=channelout  nInputs=dspba_internal_get_channel_ports(gcb)  nOutputs=dspba_internal_get_channel_ports(gcb)  omode=Inherit via internal rule  otype=sfix(16)  scale=2^-15  rndmethod=Unbiased  factor=1  satmethod=Symmetric  shift_vec=[0 1 2 -1]  value=2  inPortNames=['v'; 'c'; '0'; '1'; '2'; '3'; '4'; '5'; '6'; '7'; '8'; '9'; 'A'; 'B'; 'D'; 'E'; 'F'; 'G'; 'H'; 'I'; 'J'; 'K'; 'L'; 'M'; 'N'; 'O'; 'P'; 'Q'; 'R'; 'S'; 'T'; 'U'; 'W'; 'X'; 'Y'; 'Z']  outPortNames=['v'; 'c'; '0'; '1'; '2'; '3'; '4'; '5'; '6'; '7'; '8'; '9'; 'A'; 'B'; 'D'; 'E'; 'F'; 'G'; 'H'; 'I'; 'J'; 'K'; 'L'; 'M'; 'N'; 'O'; 'P'; 'Q'; 'R'; 'S'; 'T'; 'U'; 'W'; 'X'; 'Y'; 'Z']  dspbaimage=dspba_prim.jpg  text=fprintf('Out%s', AdvDSPBChannelOutDisplay(latency));  style=Optimised  dataSignals=2  foldingEnabled=off  channels=1  sampleRate=200  packetBeginPresent=off  packetBeginEnabled=off  visibilities=dspba_ChannelOutVis(gcb)  latency=15  latencyCorrection=0  version=20141013
  Const : DSPBAPrim/Const  primtype=const  nInputs=0  nOutputs=1  omode=Specify via dialog  otype=uint(8)  scale=0  rndmethod=Unbiased  factor=1  satmethod=Symmetric  shift_vec=[0 1 2 -1]  value=0  inPortNames=['+'; '+';]  outPortNames=[' ']  dspbaimage=dspba_prim.jpg  text=fprintf('%s', num2str(value));  style=Optimised  visibilities=8 + 1024  floatPrecision=float32_m23  version=20120820
  Const1 : DSPBAPrim/Const  primtype=const  nInputs=0  nOutputs=1  omode=Specify via dialog  otype=sfix(16)  scale=2^-15  rndmethod=Unbiased  factor=1  satmethod=Symmetric  shift_vec=[0 1 2 -1]  value=63308  inPortNames=['+'; '+';]  outPortNames=[' ']  dspbaimage=dspba_prim.jpg  text=fprintf('%s', num2str(value));  style=Optimised  visibilities=8 + 1024  floatPrecision=float32_m23  version=20120820
  Const2 : DSPBAPrim/Const  primtype=const  nInputs=0  nOutputs=1  omode=Specify via dialog  otype=sfix(16)  scale=2^-15  rndmethod=Unbiased  factor=1  satmethod=Symmetric  shift_vec=[0 1 2 -1]  value=65461  inPortNames=['+'; '+';]  outPortNames=[' ']  dspbaimage=dspba_prim.jpg  text=fprintf('%s', num2str(value));  style=Optimised  visibilities=8 + 1024  floatPrecision=float32_m23  version=20120820
  Const3 : DSPBAPrim/Const  primtype=const  nInputs=0  nOutputs=1  omode=Specify via dialog  otype=sfix(16)  scale=2^-15  rndmethod=Unbiased  factor=1  satmethod=Symmetric  shift_vec=[0 1 2 -1]  value=7320  inPortNames=['+'; '+';]  outPortNames=[' ']  dspbaimage=dspba_prim.jpg  text=fprintf('%s', num2str(value));  style=Optimised  visibilities=8 + 1024  floatPrecision=float32_m23  version=20120820
  Const4 : DSPBAPrim/Const  primtype=const  nInputs=0  nOutputs=1  omode=Specify via dialog  otype=sfix(16)  scale=2^-15  rndmethod=Unbiased  factor=1  satmethod=Symmetric  shift_vec=[0 1 2 -1]  value=7592  inPortNames=['+'; '+';]  outPortNames=[' ']  dspbaimage=dspba_prim.jpg  text=fprintf('%s', num2str(value));  style=Optimised  visibilities=8 + 1024  floatPrecision=float32_m23  version=20120820
  Const5 : DSPBAPrim/Const  primtype=const  nInputs=0  nOutputs=1  omode=Specify via dialog  otype=sfix(16)  scale=2^-15  rndmethod=Unbiased  factor=1  satmethod=Symmetric  shift_vec=[0 1 2 -1]  value=57545  inPortNames=['+'; '+';]  outPortNames=[' ']  dspbaimage=dspba_prim.jpg  text=fprintf('%s', num2str(value));  style=Optimised  visibilities=8 + 1024  floatPrecision=float32_m23  version=20120820
  Const6 : DSPBAPrim/Const  primtype=const  nInputs=0  nOutputs=1  omode=Specify via dialog  otype=sfix(16)  scale=2^-15  rndmethod=Unbiased  factor=1  satmethod=Symmetric  shift_vec=[0 1 2 -1]  value=53297  inPortNames=['+'; '+';]  outPortNames=[' ']  dspbaimage=dspba_prim.jpg  text=fprintf('%s', num2str(value));  style=Optimised  visibilities=8 + 1024  floatPrecision=float32_m23  version=20120820
  Convert{,1..7} (8 alike) : DSPBAPrim/Convert  primtype=convert  nInputs=1  nOutputs=1  omode=Specify via dialog  otype=sfix(16)  scale=2^-15  rndmethod=Unbiased  factor=1  satmethod=None  shift_vec=[0 1 2 -1]  value=round([0:255]/17)  inPortNames=[' '; ' ';]  outPortNames=[' '; 'c']  dspbaimage=dspba_prim.jpg  text=fprintf('convert');  style=Optimised  visibilities=8+64+256+2^17  clipdetect=off  floatPrecision=float32_m23  advOptions=[]  version=20130211
  Mult{,1..18} (19 alike) : DSPBAPrim/Mult  primtype=mult  nInputs=2  nOutputs=1  omode=Inherit via internal rule  otype=sfix(16)  scale=2^-15  rndmethod=Unbiased  factor=1  satmethod=Symmetric  shift_vec=[0 1 2 -1]  value=0  inPortNames=[' '; ' ';]  outPortNames=[' ']  dspbaimage=dspba_prim.jpg  text=fprintf('X');  style=Optimised  visibilities=8+2^18+2^19  floatPrecision=float32_m23  floatRounding=correct  advOptions=[]  version=20130115
  Sub : DSPBAPrim/Sub  primtype=sub  nInputs=2  nOutputs=1  omode=Inherit via internal rule with word growth  otype=sfix(16)  scale=2^-15  rndmethod=Unbiased  factor=1  satmethod=Symmetric  shift_vec=[0 1 2 -1]  value=0  inPortNames=['+'; '-';]  outPortNames=[' ']  dspbaimage=dspba_prim.jpg  text=fprintf('-');  style=Optimised  visibilities=8+2^17+2^18  floatRounding=correct  advOptions=[]  version=20130115
  Sub1 : DSPBAPrim/Sub  primtype=sub  nInputs=2  nOutputs=1  omode=Inherit via internal rule with word growth  otype=sfix(16)  scale=2^-15  rndmethod=Unbiased  factor=1  satmethod=Symmetric  shift_vec=[0 1 2 -1]  value=0  inPortNames=['+'; '-';]  outPortNames=[' ']  dspbaimage=dspba_prim.jpg  text=fprintf('-');  style=Optimised  visibilities=8+2^17+2^18  floatRounding=correct  advOptions=[]  version=20130115
  Sub2 : DSPBAPrim/Sub  primtype=sub  nInputs=2  nOutputs=1  omode=Inherit via internal rule with word growth  otype=sfix(16)  scale=2^-15  rndmethod=Unbiased  factor=1  satmethod=Symmetric  shift_vec=[0 1 2 -1]  value=0  inPortNames=['+'; '-';]  outPortNames=[' ']  dspbaimage=dspba_prim.jpg  text=fprintf('-');  style=Optimised  visibilities=8+2^17+2^18  floatRounding=correct  advOptions=[]  version=20130115
  SynthesisInfo : DSPBAPrim/SynthesisInfo  primtype=synthinfo  nInputs=0  nOutputs=0  omode=Inherit via internal rule  otype=sfix(16)  scale=2^-15  rndmethod=Truncate  factor=1  satmethod=Symmetric  shift_vec=[0 1 2 -1]  value=99  inPortNames=[' '; ' ';]  outPortNames=[' ']  dspbaimage=dspba_prim_ctrl.jpg  text=fprintf('Style=%s', style);  style=Scheduled  visibilities=2^15+2^17+2^18+2^19  constraintInUse=off  constraintRelation=>  constraintLimit=2  bitAccurate=off  version=20150220
  Terminator : Terminator
  iq_squr_real_q_out : Outport
  iq_squr_imag_q_out1 : Outport  Port=2
  iq_squr_v_out : Outport  Port=3
  iq_squr_c_out : Outport  Port=4
  wires:
  Mult/1 -> Add/1
  Mult1/1 -> Add/2
  iq_squr_imag_q_in/1 -> ChannelIn/4
  iq_squr_real_q_in/1 -> ChannelIn/3
  ChannelOut/3 -> iq_squr_real_q_out/1
  ChannelOut/1 -> iq_squr_v_out/1
  ChannelOut/2 -> iq_squr_c_out/1
  iq_squr_v_in/1 -> ChannelIn/1
  iq_squr_c_in/1 -> ChannelIn/2
  ChannelIn/2 -> Terminator/1
  ChannelIn/3 -> Mult13/1, Mult2/1, Mult8/1, Mult4/1, Mult/2, Mult/1
  ChannelIn/4 -> Mult14/1, Mult3/1, Mult5/2, Mult9/2, Mult1/2, Mult1/1
  Const/1 -> ChannelOut/2
  Add/1 -> Convert/1
  Const3/1 -> Mult16/2, Mult6/2
  Const4/1 -> Mult15/2, Mult7/2
  Mult4/1 -> Convert1/1
  Mult5/1 -> Convert2/1
  Const5/1 -> Mult18/2, Mult10/2
  Const6/1 -> Mult17/2, Mult11/2
  Mult8/1 -> Convert4/1
  Mult9/1 -> Convert5/1
  Mult12/1 -> Convert3/1
  Convert/1 -> Mult12/2, Mult12/1, Mult5/1, Mult4/2
  Convert1/1 -> Mult15/1, Mult6/1
  Convert2/1 -> Mult16/1, Mult7/1
  Convert3/1 -> Mult9/1, Mult8/2
  Convert4/1 -> Mult17/1, Mult10/1
  Convert5/1 -> Mult18/1, Mult11/1
  Add1/1 -> Convert6/1
  Add2/1 -> Convert7/1
  ChannelIn/1 -> ChannelOut/1
  Convert6/1 -> ChannelOut/3
  Convert7/1 -> ChannelOut/4
  ChannelOut/4 -> iq_squr_imag_q_out1/1
  Const1/1 -> Mult14/2, Mult2/2
  Const2/1 -> Mult13/2, Mult3/2
  Mult2/1 -> Sub/1
  Mult3/1 -> Sub/2
  Mult13/1 -> Add3/1
  Mult14/1 -> Add3/2
  Sub/1 -> Add1/1
  Add3/1 -> Add2/1
  Mult6/1 -> Sub1/1
  Mult7/1 -> Sub1/2
  Mult15/1 -> Add4/1
  Mult16/1 -> Add4/2
  Sub1/1 -> Add1/2
  Add4/1 -> Add2/2
  Mult10/1 -> Sub2/1
  Mult11/1 -> Sub2/2
  Mult17/1 -> Add5/1
  Mult18/1 -> Add5/2
  Add5/1 -> Add2/3
  Sub2/1 -> Add1/3
